simulink library "XtalkCancellation"  (R2022b)
settings: Solver=VariableStepAuto  StartTime=0.0  StopTime=10.0  RelTol=1e-3
values from neighbouring files (symbols this model uses):
  XtalkCancellationConfig = struct('IIR', IIR,                                       'numFilters', numFilters,                                       'numHeadrests', numHeadrests,                                      'numFilterPerSpkr', numFilterPerSpkr,                                      'frameSize', frameSize,                                       'maxDelayPool', maxDelayPool,                                      'delayDe ...(+21 chars)    [XtalkCancellationInit.m]
undefined symbols (not defined in the file or in its folder): repelem
libraries: FeaturePath x1, PoolDelay x1, PooliirLib x1, TuneVar x1
settings Model: Creator=ud1041536  LastModifiedBy=sc48041
settings SolverCC: AlgebraicLoopSolver=TrustRegion
settings DataIOCC: ReturnWorkspaceOutputs=off
settings DebuggingCC: UnconnectedInputMsg=warning  UnconnectedOutputMsg=warning  UnconnectedLineMsg=warning  SFMachineParentedDataDiag=warning  ArithmeticOperatorsInVariantConditions=warning
settings ModelReferenceCC: EnableRefExpFcnMdlSchedulingChecks=on
settings SFSimCC: CustomCodeUndefinedFunction=UseInterfaceOnly

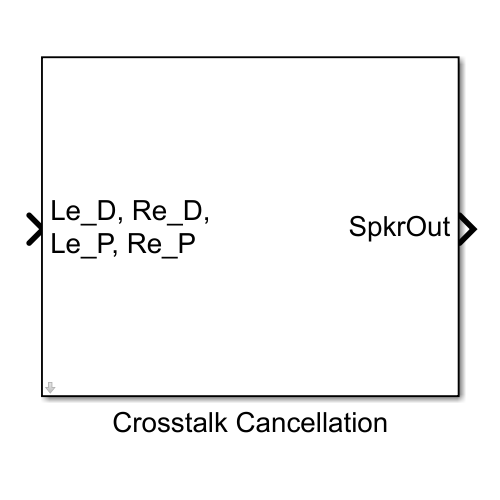
[thumbnail: Simulink's stored preview of the top-level diagram]
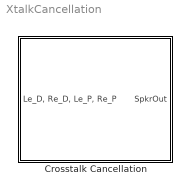
== system XtalkCancellation ==
  Crosstalk Cancellation : Subsystem  mask{configStruct=XtalkCancellationConfig}
      mask prompts: configStruct "Config struct name:"
      mask init:
      | IIR = configStruct.IIR;
      mask Display:
      | port_label('input', 1, sprintf('Le_D, Re_D,\nLe_P, Re_P'));
      | port_label('output', 1, 'SpkrOut');

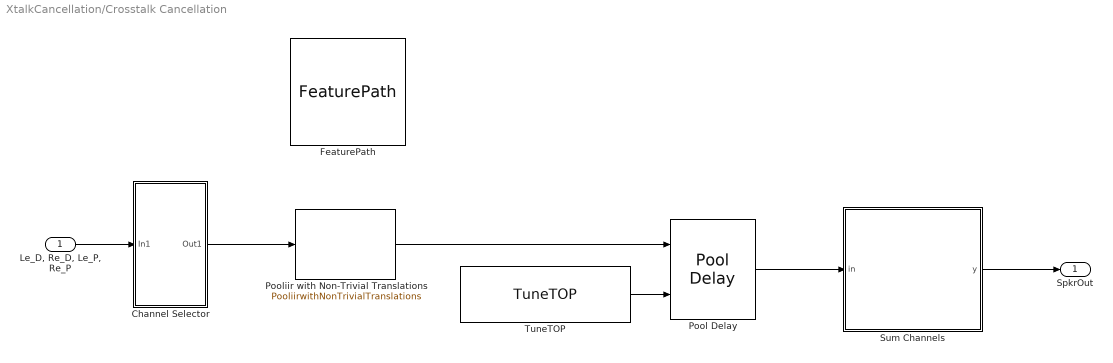
== system XtalkCancellation/Crosstalk Cancellation ==
  "Le_D, Re_D, Le_P, Re_P" : Inport
  Channel Selector : Subsystem
  FeaturePath : FeaturePath/FeaturePath  FeatureName=XtalkCancellation  IsGroup=off  GroupNumber=-1  IsModule=off  TriggerInit=[365 -126 480 -19]
      settings: SourceProductName=Bose Talaria
  Pool Delay : PoolDelay/Pool Delay  maxTotalDelay=configStruct.maxDelayPool  frameSize=configStruct.frameSize  numChannels=configStruct.numFilters  bufferAlias=[]  headerFilename=[]
  Pooliir with Non-Trivial Translations : PooliirLib/PooliirwithNonTrivialTranslations  maxNumStages=IIR.maxNumStages  numStages=IIR.numStages  sosCoefficients=IIR.coeffs  alias=IIR.alias  variantType=IIR.variantSelect  FeatureName=IIR
  Sum Channels : MATLAB Function  Priority=3  TreatAsAtomicUnit=on
  TuneTOP : TuneVar/TuneTOP  TriggerInit=[535 102 705 158]  TopName=Delay  TuneName=Delay  DataTypeOut=int32  TunabilityNumber=1  MinValue=[]  MaxValue=[]  BankNumber=0  PreOverlay=false  PostOverlay=false  UseSameName=on  MaskValue=configStruct.delayDefault
      settings: SourceProductName=Bose Talaria
  SpkrOut : Outport  VectorParamsAs1DForOutWhenUnconnected=off
  wires:
  Pooliir with Non-Trivial Translations/1 -> Pool Delay/1
  Pool Delay/1 -> Sum Channels/1(in)
  TuneTOP/1 -> Pool Delay/2
  Sum Channels/1(y) -> SpkrOut/1
  Channel Selector/1(Out1) -> Pooliir with Non-Trivial Translations/1
  "Le_D, Re_D, Le_P, Re_P"/1 -> Channel Selector/1(In1)

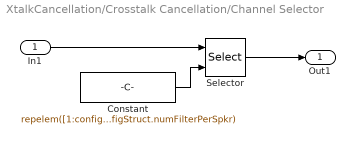
== system XtalkCancellation/Crosstalk Cancellation/Channel Selector ==
  In1 : Inport
  Constant : Constant  Value=repelem([1:configStruct.numHeadrests], configStruct.numFilterPerSpkr)
  Selector : Selector  NumberOfDimensions=2  InputPortWidth=3  IndexOptions=Select all,Index vector (port)  Indices=[1 3],1  OutputSizes=1,1
  Out1 : Outport  VectorParamsAs1DForOutWhenUnconnected=off
  wires:
  Constant/1 -> Selector/2
  Selector/1 -> Out1/1
  In1/1 -> Selector/1

== matlab function XtalkCancellation/Crosstalk Cancellation/Sum Channels ==
  data: in input; y output; configStruct parameter
function y = sumChannels(in, configStruct)

numFilters = configStruct.numFilters;
numHeadrests = configStruct.numHeadrests;
numFilterPerSpkr = configStruct.numFilterPerSpkr;

[frameSize, ~] = size(in);
y = coder.nullcopy(single(zeros(frameSize, numHeadrests)));

for i = 1:numHeadrests
    y(:,i) = sum(in(:,i:numFilterPerSpkr:numFilters),2);
end
